simulink model "pd_path_sg"  (R2013b)
settings: Solver=ode45  StartTime=0.0  StopTime=10  RelTol=1e-3
undefined symbols (not defined in the file or in its folder): A, A2, B, C, D, EVAL, i, output_samp_bcoef, PCIN, reg_pk_lim, reg_plim, reg_scale, reg_sr_lim, reg_staclr, reg_txgain, THIS_DATE, W, X, Z
undefined symbols (not defined in the file): lut_address, lut_address_s5, reg_dltap
libraries: xbsIndex_r4 x3819, lut_ram_vhdl x32
(part 13 of 31)

== system pd_path_sg/A_lut_store/one_lut1/interp_a0 ==
  b0 : Inport
  b1 : Inport  Port=2
  delta : Inport  Port=3
  Convert : xbsIndex_r4/Convert  gui_display_data_type=Fixed-point  arith_type="Signed  (2's comp)"  n_bits=30  bin_pt=0  float_type=Single  exp_bits=8  fraction_bits=24  quantization=Truncate  overflow=Wrap  en=off  latency=0  pipeline=off  dbl_ovrd=off  block_type=convert
  Convert1 : xbsIndex_r4/Convert  gui_display_data_type=Fixed-point  arith_type="Signed  (2's comp)"  n_bits=48  bin_pt=0  float_type=Single  exp_bits=8  fraction_bits=24  quantization=Truncate  overflow=Wrap  en=off  latency=0  pipeline=off  dbl_ovrd=off  block_type=convert
  Convert2 : xbsIndex_r4/Convert  gui_display_data_type=Fixed-point  arith_type="Signed  (2's comp)"  n_bits=18  bin_pt=0  float_type=Single  exp_bits=8  fraction_bits=24  quantization=Truncate  overflow=Wrap  en=off  latency=0  pipeline=off  dbl_ovrd=off  block_type=convert
  Convert3 : xbsIndex_r4/Convert  gui_display_data_type=Fixed-point  arith_type="Signed  (2's comp)"  n_bits=27  bin_pt=0  float_type=Single  exp_bits=8  fraction_bits=24  quantization=Truncate  overflow=Wrap  en=off  latency=0  pipeline=off  dbl_ovrd=off  block_type=convert
  Convert4 : xbsIndex_r4/Convert  gui_display_data_type=Fixed-point  arith_type="Signed  (2's comp)"  n_bits=30  bin_pt=0  float_type=Single  exp_bits=8  fraction_bits=24  quantization=Truncate  overflow=Wrap  en=off  latency=0  pipeline=off  dbl_ovrd=off  block_type=convert
  Convert5 : xbsIndex_r4/Convert  gui_display_data_type=Fixed-point  arith_type="Signed  (2's comp)"  n_bits=18  bin_pt=0  float_type=Single  exp_bits=8  fraction_bits=24  quantization=Truncate  overflow=Wrap  en=off  latency=0  pipeline=off  dbl_ovrd=off  block_type=convert
  Convert6 : xbsIndex_r4/Convert  gui_display_data_type=Fixed-point  arith_type="Signed  (2's comp)"  n_bits=48  bin_pt=0  float_type=Single  exp_bits=8  fraction_bits=24  quantization=Truncate  overflow=Wrap  en=off  latency=0  pipeline=off  dbl_ovrd=off  block_type=convert
  Convert7 : xbsIndex_r4/Convert  gui_display_data_type=Fixed-point  arith_type="Signed  (2's comp)"  n_bits=27  bin_pt=0  float_type=Single  exp_bits=8  fraction_bits=24  quantization=Truncate  overflow=Wrap  en=off  latency=0  pipeline=off  dbl_ovrd=off  block_type=convert
  Convert8 : xbsIndex_r4/Convert  gui_display_data_type=Fixed-point  arith_type="Signed  (2's comp)"  n_bits=22  bin_pt=0  float_type=Single  exp_bits=8  fraction_bits=24  quantization=Truncate  overflow=Wrap  en=off  latency=0  pipeline=off  dbl_ovrd=off  block_type=convert
  Convert9 : xbsIndex_r4/Convert  gui_display_data_type=Fixed-point  arith_type="Signed  (2's comp)"  n_bits=22  bin_pt=0  float_type=Single  exp_bits=8  fraction_bits=24  quantization=Truncate  overflow=Wrap  en=off  latency=0  pipeline=off  dbl_ovrd=off  block_type=convert
  "DSP48E2 " : xbsIndex_r4/DSP48E2   use_a=Direct from A Port  use_b=Direct from B Port  addsub_mode=ONE48  xl_useadderonly=off  xl_dynamicmult=off  preaddinsel=A  amultsel=AD  bmultsel=B  enable_d=on  reset_preg=off  auto_reset_pr=RESET  pattern_from_creg=1  pattern='000000000000'  mask_from_creg=1  pattern_mask='000000000000'  rnd='000000000000'  widexor=off  xormode=1  use_op=on  use_creg=on  rst_all=off  en_all=off  use_pcin=off  use_carrycascin=off  use_multsignin=off  use_carryout=off  use_patterndetect=off  use_patternbdetect=off  use_overflow=off  use_underflow=off  use_acout=off  use_bcout=off  use_pcout=off  use_multsignout=off  use_carrycascout=off  pipeline_a=1  pipeline_b=2  pipeline_acout=1  pipeline_bcout=1  pipeline_c=on  pipeline_p=on  pipeline_mult=on  pipeline_opmode=on  pipeline_alumode=on  pipeline_carryin=on  pipeline_carryinsel=on  dreg=on  adreg=on  register_inmode=off  rst_a=off  rst_b=off  rst_c=off  rst_mult=off  rst_p=off  rst_carry_in=off  rst_alumode=off  rst_ctrl=off  reset_port_d=off  reset_port_inmode=off  en_a1=off  en_a2=off  en_b1=off  en_b2=off  en_c=off  en_mult=off  en_p=off  en_carry_in=off  en_alumode=off  en_multcarryin=off  en_ctrl=off  enable_port_regd=off  enable_port_regad=off  enable_port_reginmode=off  alumode_inverted=off  alumode_inverted_value='0000'  is_carryin_inverted=off  inmode_inverted=off  inmode_inverted_value='00000'  opmode_inverted=off  opmode_inverted_value='000000000'  is_rstallcarryin_inverted=off  is_rstalumode_inverted=off  is_rsta_inverted=off  is_rstb_inverted=off  is_rstc_inverted=off  is_rstd_inverted=off  is_rstctrl_inverted=off  is_rstinmode_inverted=off  is_rstm_inverted=off  is_rstp_inverted=off  use_synth_model=off  is_clk_inverted=false  block_type=dsp48e2
  DSP48E2 1 : xbsIndex_r4/DSP48E2   use_a=Direct from A Port  use_b=Direct from B Port  addsub_mode=ONE48  xl_useadderonly=off  xl_dynamicmult=off  preaddinsel=A  amultsel=AD  bmultsel=B  enable_d=on  reset_preg=off  auto_reset_pr=RESET  pattern_from_creg=1  pattern='000000000000'  mask_from_creg=1  pattern_mask='000000000000'  rnd='000000000000'  widexor=off  xormode=1  use_op=on  use_creg=on  rst_all=off  en_all=off  use_pcin=off  use_carrycascin=off  use_multsignin=off  use_carryout=off  use_patterndetect=off  use_patternbdetect=off  use_overflow=off  use_underflow=off  use_acout=off  use_bcout=off  use_pcout=off  use_multsignout=off  use_carrycascout=off  pipeline_a=1  pipeline_b=2  pipeline_acout=1  pipeline_bcout=1  pipeline_c=on  pipeline_p=on  pipeline_mult=on  pipeline_opmode=on  pipeline_alumode=on  pipeline_carryin=on  pipeline_carryinsel=on  dreg=on  adreg=on  register_inmode=off  rst_a=off  rst_b=off  rst_c=off  rst_mult=off  rst_p=off  rst_carry_in=off  rst_alumode=off  rst_ctrl=off  reset_port_d=off  reset_port_inmode=off  en_a1=off  en_a2=off  en_b1=off  en_b2=off  en_c=off  en_mult=off  en_p=off  en_carry_in=off  en_alumode=off  en_multcarryin=off  en_ctrl=off  enable_port_regd=off  enable_port_regad=off  enable_port_reginmode=off  alumode_inverted=off  alumode_inverted_value='0000'  is_carryin_inverted=off  inmode_inverted=off  inmode_inverted_value='00000'  opmode_inverted=off  opmode_inverted_value='000000000'  is_rstallcarryin_inverted=off  is_rstalumode_inverted=off  is_rsta_inverted=off  is_rstb_inverted=off  is_rstc_inverted=off  is_rstd_inverted=off  is_rstctrl_inverted=off  is_rstinmode_inverted=off  is_rstm_inverted=off  is_rstp_inverted=off  use_synth_model=off  is_clk_inverted=false  block_type=dsp48e2
  Delay : xbsIndex_r4/Delay  rst=off  infoeditControl=Selection of Reset will increase slice count due to use of real FFs and instead of SRLs  en=off  latency=2  reg_retiming=off  dbl_ovrd=off  block_type=delay
      settings: infoedit=Hardware notes: A delay line is a chain, each link of which is an SRL16 or SRL32 followed by a flip-flop.
  Delay1 : xbsIndex_r4/Delay  rst=off  infoeditControl=Selection of Reset will increase slice count due to use of real FFs and instead of SRLs  en=off  latency=2  reg_retiming=off  dbl_ovrd=off  block_type=delay
      settings: infoedit=Hardware notes: A delay line is a chain, each link of which is an SRL16 or SRL32 followed by a flip-flop.
  Delay2 : xbsIndex_r4/Delay  rst=off  infoeditControl=Selection of Reset will increase slice count due to use of real FFs and instead of SRLs  en=off  latency=1  reg_retiming=off  dbl_ovrd=off  block_type=delay
      settings: infoedit=Hardware notes: A delay line is a chain, each link of which is an SRL16 or SRL32 followed by a flip-flop.
  Delay3 : xbsIndex_r4/Delay  rst=off  infoeditControl=Selection of Reset will increase slice count due to use of real FFs and instead of SRLs  en=off  latency=1  reg_retiming=off  dbl_ovrd=off  block_type=delay
      settings: infoedit=Hardware notes: A delay line is a chain, each link of which is an SRL16 or SRL32 followed by a flip-flop.
  Demux : Demux  Outputs=2
  Demux1 : Demux  Outputs=2
  Mux : Mux  Inputs=2
  Opmode : xbsIndex_r4/Opmode  device=DSP48E2  equ=P=C+(A*B)  operation=C + A*B  inmode_0_3=D-A2  inmode_1_3=(D-A)*B  preaddinsel=A  amultsel=AD  bmultsel=B  inmode_0=A2  inmode_4=B2  logicinstr=X XOR Z  z_mux=PCIN>>17  xy_mux=P  w_mux=P  carry=CIN  dbl_ovrd=off  operand=+  x_mux=P  block_type=opmode
  Opmode1 : xbsIndex_r4/Opmode  device=DSP48E2  equ=P=C+(A*B)  operation=C + A*B  inmode_0_3=D-A2  inmode_1_3=(D-A)*B  preaddinsel=A  amultsel=AD  bmultsel=B  inmode_0=A2  inmode_4=B2  logicinstr=X XOR Z  z_mux=PCIN>>17  xy_mux=P  w_mux=P  carry=CIN  dbl_ovrd=off  operand=+  x_mux=P  block_type=opmode
  Reinterpret{,1..7} (8 alike) : xbsIndex_r4/Reinterpret  force_arith_type=on  arith_type="Signed  (2's comp)"  force_bin_pt=on  bin_pt=0  block_type=reinterpret
  Shift : xbsIndex_r4/Shift  shift_dir=Left  shift_bits=6  en=off  latency=0  precision=Full  arith_type="Signed  (2's comp)"  n_bits=16  bin_pt=14  quantization=Truncate  overflow=Wrap  dbl_ovrd=off  block_type=shift
  Shift1 : xbsIndex_r4/Shift  shift_dir=Left  shift_bits=6  en=off  latency=0  precision=Full  arith_type="Signed  (2's comp)"  n_bits=16  bin_pt=14  quantization=Truncate  overflow=Wrap  dbl_ovrd=off  block_type=shift
  q : Outport
  wires:
  Shift1/1 -> DSP48E2 1/3
  Shift/1 -> "DSP48E2 "/3
  Delay/1 -> Reinterpret1/1
  Delay1/1 -> Reinterpret6/1
  Mux/1 -> q/1
  "DSP48E2 "/1 -> Convert8/1
  Opmode1/1 -> "DSP48E2 "/5
  Convert7/1 -> "DSP48E2 "/4
  Reinterpret7/1 -> Convert7/1
  Convert6/1 -> Shift/1
  Reinterpret6/1 -> Convert6/1
  Convert5/1 -> "DSP48E2 "/2
  Reinterpret5/1 -> Convert5/1
  Convert4/1 -> "DSP48E2 "/1
  Reinterpret4/1 -> Convert4/1
  delta/1 -> Reinterpret2/1, Reinterpret5/1
  b1/1 -> Demux1/1
  b0/1 -> Demux/1
  Convert9/1 -> Delay3/1
  Reinterpret3/1 -> Convert3/1
  Convert3/1 -> DSP48E2 1/4
  Reinterpret2/1 -> Convert2/1
  Convert2/1 -> DSP48E2 1/2
  Reinterpret1/1 -> Convert1/1
  Convert1/1 -> Shift1/1
  Convert/1 -> DSP48E2 1/1
  Reinterpret/1 -> Convert/1
  Opmode/1 -> DSP48E2 1/5
  DSP48E2 1/1 -> Convert9/1
  Delay2/1 -> Mux/1  "I"
  Convert8/1 -> Delay2/1
  Delay3/1 -> Mux/2  "Q"
  Demux/1 -> Delay1/1, Reinterpret4/1
  Demux/2 -> Reinterpret/1, Delay/1
  Demux1/1 -> Reinterpret7/1
  Demux1/2 -> Reinterpret3/1

== system pd_path_sg/A_lut_store/one_lut1/interp_a1 ==
  b0 : Inport
  b1 : Inport  Port=2
  delta : Inport  Port=3
  Convert : xbsIndex_r4/Convert  gui_display_data_type=Fixed-point  arith_type="Signed  (2's comp)"  n_bits=30  bin_pt=0  float_type=Single  exp_bits=8  fraction_bits=24  quantization=Truncate  overflow=Wrap  en=off  latency=0  pipeline=off  dbl_ovrd=off  block_type=convert
  Convert1 : xbsIndex_r4/Convert  gui_display_data_type=Fixed-point  arith_type="Signed  (2's comp)"  n_bits=48  bin_pt=0  float_type=Single  exp_bits=8  fraction_bits=24  quantization=Truncate  overflow=Wrap  en=off  latency=0  pipeline=off  dbl_ovrd=off  block_type=convert
  Convert2 : xbsIndex_r4/Convert  gui_display_data_type=Fixed-point  arith_type="Signed  (2's comp)"  n_bits=18  bin_pt=0  float_type=Single  exp_bits=8  fraction_bits=24  quantization=Truncate  overflow=Wrap  en=off  latency=0  pipeline=off  dbl_ovrd=off  block_type=convert
  Convert3 : xbsIndex_r4/Convert  gui_display_data_type=Fixed-point  arith_type="Signed  (2's comp)"  n_bits=27  bin_pt=0  float_type=Single  exp_bits=8  fraction_bits=24  quantization=Truncate  overflow=Wrap  en=off  latency=0  pipeline=off  dbl_ovrd=off  block_type=convert
  Convert4 : xbsIndex_r4/Convert  gui_display_data_type=Fixed-point  arith_type="Signed  (2's comp)"  n_bits=30  bin_pt=0  float_type=Single  exp_bits=8  fraction_bits=24  quantization=Truncate  overflow=Wrap  en=off  latency=0  pipeline=off  dbl_ovrd=off  block_type=convert
  Convert5 : xbsIndex_r4/Convert  gui_display_data_type=Fixed-point  arith_type="Signed  (2's comp)"  n_bits=18  bin_pt=0  float_type=Single  exp_bits=8  fraction_bits=24  quantization=Truncate  overflow=Wrap  en=off  latency=0  pipeline=off  dbl_ovrd=off  block_type=convert
  Convert6 : xbsIndex_r4/Convert  gui_display_data_type=Fixed-point  arith_type="Signed  (2's comp)"  n_bits=48  bin_pt=0  float_type=Single  exp_bits=8  fraction_bits=24  quantization=Truncate  overflow=Wrap  en=off  latency=0  pipeline=off  dbl_ovrd=off  block_type=convert
  Convert7 : xbsIndex_r4/Convert  gui_display_data_type=Fixed-point  arith_type="Signed  (2's comp)"  n_bits=27  bin_pt=0  float_type=Single  exp_bits=8  fraction_bits=24  quantization=Truncate  overflow=Wrap  en=off  latency=0  pipeline=off  dbl_ovrd=off  block_type=convert
  Convert8 : xbsIndex_r4/Convert  gui_display_data_type=Fixed-point  arith_type="Signed  (2's comp)"  n_bits=22  bin_pt=0  float_type=Single  exp_bits=8  fraction_bits=24  quantization=Truncate  overflow=Wrap  en=off  latency=0  pipeline=off  dbl_ovrd=off  block_type=convert
  Convert9 : xbsIndex_r4/Convert  gui_display_data_type=Fixed-point  arith_type="Signed  (2's comp)"  n_bits=22  bin_pt=0  float_type=Single  exp_bits=8  fraction_bits=24  quantization=Truncate  overflow=Wrap  en=off  latency=0  pipeline=off  dbl_ovrd=off  block_type=convert
  "DSP48E2 " : xbsIndex_r4/DSP48E2   use_a=Direct from A Port  use_b=Direct from B Port  addsub_mode=ONE48  xl_useadderonly=off  xl_dynamicmult=off  preaddinsel=A  amultsel=AD  bmultsel=B  enable_d=on  reset_preg=off  auto_reset_pr=RESET  pattern_from_creg=1  pattern='000000000000'  mask_from_creg=1  pattern_mask='000000000000'  rnd='000000000000'  widexor=off  xormode=1  use_op=on  use_creg=on  rst_all=off  en_all=off  use_pcin=off  use_carrycascin=off  use_multsignin=off  use_carryout=off  use_patterndetect=off  use_patternbdetect=off  use_overflow=off  use_underflow=off  use_acout=off  use_bcout=off  use_pcout=off  use_multsignout=off  use_carrycascout=off  pipeline_a=1  pipeline_b=2  pipeline_acout=1  pipeline_bcout=1  pipeline_c=on  pipeline_p=on  pipeline_mult=on  pipeline_opmode=on  pipeline_alumode=on  pipeline_carryin=on  pipeline_carryinsel=on  dreg=on  adreg=on  register_inmode=off  rst_a=off  rst_b=off  rst_c=off  rst_mult=off  rst_p=off  rst_carry_in=off  rst_alumode=off  rst_ctrl=off  reset_port_d=off  reset_port_inmode=off  en_a1=off  en_a2=off  en_b1=off  en_b2=off  en_c=off  en_mult=off  en_p=off  en_carry_in=off  en_alumode=off  en_multcarryin=off  en_ctrl=off  enable_port_regd=off  enable_port_regad=off  enable_port_reginmode=off  alumode_inverted=off  alumode_inverted_value='0000'  is_carryin_inverted=off  inmode_inverted=off  inmode_inverted_value='00000'  opmode_inverted=off  opmode_inverted_value='000000000'  is_rstallcarryin_inverted=off  is_rstalumode_inverted=off  is_rsta_inverted=off  is_rstb_inverted=off  is_rstc_inverted=off  is_rstd_inverted=off  is_rstctrl_inverted=off  is_rstinmode_inverted=off  is_rstm_inverted=off  is_rstp_inverted=off  use_synth_model=off  is_clk_inverted=false  block_type=dsp48e2
  DSP48E2 1 : xbsIndex_r4/DSP48E2   use_a=Direct from A Port  use_b=Direct from B Port  addsub_mode=ONE48  xl_useadderonly=off  xl_dynamicmult=off  preaddinsel=A  amultsel=AD  bmultsel=B  enable_d=on  reset_preg=off  auto_reset_pr=RESET  pattern_from_creg=1  pattern='000000000000'  mask_from_creg=1  pattern_mask='000000000000'  rnd='000000000000'  widexor=off  xormode=1  use_op=on  use_creg=on  rst_all=off  en_all=off  use_pcin=off  use_carrycascin=off  use_multsignin=off  use_carryout=off  use_patterndetect=off  use_patternbdetect=off  use_overflow=off  use_underflow=off  use_acout=off  use_bcout=off  use_pcout=off  use_multsignout=off  use_carrycascout=off  pipeline_a=1  pipeline_b=2  pipeline_acout=1  pipeline_bcout=1  pipeline_c=on  pipeline_p=on  pipeline_mult=on  pipeline_opmode=on  pipeline_alumode=on  pipeline_carryin=on  pipeline_carryinsel=on  dreg=on  adreg=on  register_inmode=off  rst_a=off  rst_b=off  rst_c=off  rst_mult=off  rst_p=off  rst_carry_in=off  rst_alumode=off  rst_ctrl=off  reset_port_d=off  reset_port_inmode=off  en_a1=off  en_a2=off  en_b1=off  en_b2=off  en_c=off  en_mult=off  en_p=off  en_carry_in=off  en_alumode=off  en_multcarryin=off  en_ctrl=off  enable_port_regd=off  enable_port_regad=off  enable_port_reginmode=off  alumode_inverted=off  alumode_inverted_value='0000'  is_carryin_inverted=off  inmode_inverted=off  inmode_inverted_value='00000'  opmode_inverted=off  opmode_inverted_value='000000000'  is_rstallcarryin_inverted=off  is_rstalumode_inverted=off  is_rsta_inverted=off  is_rstb_inverted=off  is_rstc_inverted=off  is_rstd_inverted=off  is_rstctrl_inverted=off  is_rstinmode_inverted=off  is_rstm_inverted=off  is_rstp_inverted=off  use_synth_model=off  is_clk_inverted=false  block_type=dsp48e2
  Delay : xbsIndex_r4/Delay  rst=off  infoeditControl=Selection of Reset will increase slice count due to use of real FFs and instead of SRLs  en=off  latency=2  reg_retiming=off  dbl_ovrd=off  block_type=delay
      settings: infoedit=Hardware notes: A delay line is a chain, each link of which is an SRL16 or SRL32 followed by a flip-flop.
  Delay1 : xbsIndex_r4/Delay  rst=off  infoeditControl=Selection of Reset will increase slice count due to use of real FFs and instead of SRLs  en=off  latency=2  reg_retiming=off  dbl_ovrd=off  block_type=delay
      settings: infoedit=Hardware notes: A delay line is a chain, each link of which is an SRL16 or SRL32 followed by a flip-flop.
  Delay2 : xbsIndex_r4/Delay  rst=off  infoeditControl=Selection of Reset will increase slice count due to use of real FFs and instead of SRLs  en=off  latency=1  reg_retiming=off  dbl_ovrd=off  block_type=delay
      settings: infoedit=Hardware notes: A delay line is a chain, each link of which is an SRL16 or SRL32 followed by a flip-flop.
  Delay3 : xbsIndex_r4/Delay  rst=off  infoeditControl=Selection of Reset will increase slice count due to use of real FFs and instead of SRLs  en=off  latency=1  reg_retiming=off  dbl_ovrd=off  block_type=delay
      settings: infoedit=Hardware notes: A delay line is a chain, each link of which is an SRL16 or SRL32 followed by a flip-flop.
  Demux : Demux  Outputs=2
  Demux1 : Demux  Outputs=2
  Mux : Mux  Inputs=2
  Opmode : xbsIndex_r4/Opmode  device=DSP48E2  equ=P=C+(A*B)  operation=C + A*B  inmode_0_3=D-A2  inmode_1_3=(D-A)*B  preaddinsel=A  amultsel=AD  bmultsel=B  inmode_0=A2  inmode_4=B2  logicinstr=X XOR Z  z_mux=PCIN>>17  xy_mux=P  w_mux=P  carry=CIN  dbl_ovrd=off  operand=+  x_mux=P  block_type=opmode
  Opmode1 : xbsIndex_r4/Opmode  device=DSP48E2  equ=P=C+(A*B)  operation=C + A*B  inmode_0_3=D-A2  inmode_1_3=(D-A)*B  preaddinsel=A  amultsel=AD  bmultsel=B  inmode_0=A2  inmode_4=B2  logicinstr=X XOR Z  z_mux=PCIN>>17  xy_mux=P  w_mux=P  carry=CIN  dbl_ovrd=off  operand=+  x_mux=P  block_type=opmode
  Reinterpret{,1..7} (8 alike) : xbsIndex_r4/Reinterpret  force_arith_type=on  arith_type="Signed  (2's comp)"  force_bin_pt=on  bin_pt=0  block_type=reinterpret
  Shift : xbsIndex_r4/Shift  shift_dir=Left  shift_bits=6  en=off  latency=0  precision=Full  arith_type="Signed  (2's comp)"  n_bits=16  bin_pt=14  quantization=Truncate  overflow=Wrap  dbl_ovrd=off  block_type=shift
  Shift1 : xbsIndex_r4/Shift  shift_dir=Left  shift_bits=6  en=off  latency=0  precision=Full  arith_type="Signed  (2's comp)"  n_bits=16  bin_pt=14  quantization=Truncate  overflow=Wrap  dbl_ovrd=off  block_type=shift
  q : Outport
  wires:
  Demux1/2 -> Reinterpret3/1
  Demux1/1 -> Reinterpret7/1
  Demux/2 -> Delay/1, Reinterpret/1
  Demux/1 -> Reinterpret4/1, Delay1/1
  Delay3/1 -> Mux/2  "Q"
  Convert8/1 -> Delay2/1
  Delay2/1 -> Mux/1  "I"
  DSP48E2 1/1 -> Convert9/1
  Opmode/1 -> DSP48E2 1/5
  Reinterpret/1 -> Convert/1
  Convert/1 -> DSP48E2 1/1
  Convert1/1 -> Shift1/1
  Reinterpret1/1 -> Convert1/1
  Convert2/1 -> DSP48E2 1/2
  Reinterpret2/1 -> Convert2/1
  Convert3/1 -> DSP48E2 1/4
  Reinterpret3/1 -> Convert3/1
  Convert9/1 -> Delay3/1
  b0/1 -> Demux/1
  b1/1 -> Demux1/1
  delta/1 -> Reinterpret5/1, Reinterpret2/1
  Reinterpret4/1 -> Convert4/1
  Convert4/1 -> "DSP48E2 "/1
  Reinterpret5/1 -> Convert5/1
  Convert5/1 -> "DSP48E2 "/2
  Reinterpret6/1 -> Convert6/1
  Convert6/1 -> Shift/1
  Reinterpret7/1 -> Convert7/1
  Convert7/1 -> "DSP48E2 "/4
  Opmode1/1 -> "DSP48E2 "/5
  "DSP48E2 "/1 -> Convert8/1
  Mux/1 -> q/1
  Delay1/1 -> Reinterpret6/1
  Delay/1 -> Reinterpret1/1
  Shift/1 -> "DSP48E2 "/3
  Shift1/1 -> DSP48E2 1/3

== system pd_path_sg/A_lut_store/one_lut1/interp_b ==
  b0 : Inport
  b1 : Inport  Port=2
  delta : Inport  Port=3
  Convert : xbsIndex_r4/Convert  gui_display_data_type=Fixed-point  arith_type="Signed  (2's comp)"  n_bits=30  bin_pt=0  float_type=Single  exp_bits=8  fraction_bits=24  quantization=Truncate  overflow=Wrap  en=off  latency=0  pipeline=off  dbl_ovrd=off  block_type=convert
  Convert1 : xbsIndex_r4/Convert  gui_display_data_type=Fixed-point  arith_type="Signed  (2's comp)"  n_bits=48  bin_pt=0  float_type=Single  exp_bits=8  fraction_bits=24  quantization=Truncate  overflow=Wrap  en=off  latency=0  pipeline=off  dbl_ovrd=off  block_type=convert
  Convert10 : xbsIndex_r4/Convert  gui_display_data_type=Fixed-point  arith_type="Signed  (2's comp)"  n_bits=16  bin_pt=0  float_type=Single  exp_bits=8  fraction_bits=24  quantization=Truncate  overflow=Wrap  en=off  latency=0  pipeline=off  dbl_ovrd=off  block_type=convert
  Convert2 : xbsIndex_r4/Convert  gui_display_data_type=Fixed-point  arith_type="Signed  (2's comp)"  n_bits=18  bin_pt=0  float_type=Single  exp_bits=8  fraction_bits=24  quantization=Truncate  overflow=Wrap  en=off  latency=0  pipeline=off  dbl_ovrd=off  block_type=convert
  Convert3 : xbsIndex_r4/Convert  gui_display_data_type=Fixed-point  arith_type="Signed  (2's comp)"  n_bits=27  bin_pt=0  float_type=Single  exp_bits=8  fraction_bits=24  quantization=Truncate  overflow=Wrap  en=off  latency=0  pipeline=off  dbl_ovrd=off  block_type=convert
  Convert4 : xbsIndex_r4/Convert  gui_display_data_type=Fixed-point  arith_type="Signed  (2's comp)"  n_bits=30  bin_pt=0  float_type=Single  exp_bits=8  fraction_bits=24  quantization=Truncate  overflow=Wrap  en=off  latency=0  pipeline=off  dbl_ovrd=off  block_type=convert
  Convert5 : xbsIndex_r4/Convert  gui_display_data_type=Fixed-point  arith_type="Signed  (2's comp)"  n_bits=18  bin_pt=0  float_type=Single  exp_bits=8  fraction_bits=24  quantization=Truncate  overflow=Wrap  en=off  latency=0  pipeline=off  dbl_ovrd=off  block_type=convert
  Convert6 : xbsIndex_r4/Convert  gui_display_data_type=Fixed-point  arith_type="Signed  (2's comp)"  n_bits=48  bin_pt=0  float_type=Single  exp_bits=8  fraction_bits=24  quantization=Truncate  overflow=Wrap  en=off  latency=0  pipeline=off  dbl_ovrd=off  block_type=convert
  Convert7 : xbsIndex_r4/Convert  gui_display_data_type=Fixed-point  arith_type="Signed  (2's comp)"  n_bits=27  bin_pt=0  float_type=Single  exp_bits=8  fraction_bits=24  quantization=Truncate  overflow=Wrap  en=off  latency=0  pipeline=off  dbl_ovrd=off  block_type=convert
  Convert8 : xbsIndex_r4/Convert  gui_display_data_type=Fixed-point  arith_type="Signed  (2's comp)"  n_bits=16  bin_pt=0  float_type=Single  exp_bits=8  fraction_bits=24  quantization=Truncate  overflow=Wrap  en=off  latency=0  pipeline=off  dbl_ovrd=off  block_type=convert
  "DSP48E2 " : xbsIndex_r4/DSP48E2   use_a=Direct from A Port  use_b=Direct from B Port  addsub_mode=ONE48  xl_useadderonly=off  xl_dynamicmult=off  preaddinsel=A  amultsel=AD  bmultsel=B  enable_d=on  reset_preg=off  auto_reset_pr=RESET  pattern_from_creg=1  pattern='000000000000'  mask_from_creg=1  pattern_mask='000000000000'  rnd='000000000800'  widexor=off  xormode=1  use_op=on  use_creg=on  rst_all=off  en_all=off  use_pcin=off  use_carrycascin=off  use_multsignin=off  use_carryout=off  use_patterndetect=off  use_patternbdetect=off  use_overflow=off  use_underflow=off  use_acout=off  use_bcout=off  use_pcout=off  use_multsignout=off  use_carrycascout=off  pipeline_a=1  pipeline_b=2  pipeline_acout=1  pipeline_bcout=1  pipeline_c=on  pipeline_p=on  pipeline_mult=on  pipeline_opmode=on  pipeline_alumode=on  pipeline_carryin=on  pipeline_carryinsel=on  dreg=on  adreg=on  register_inmode=off  rst_a=off  rst_b=off  rst_c=off  rst_mult=off  rst_p=off  rst_carry_in=off  rst_alumode=off  rst_ctrl=off  reset_port_d=off  reset_port_inmode=off  en_a1=off  en_a2=off  en_b1=off  en_b2=off  en_c=off  en_mult=off  en_p=off  en_carry_in=off  en_alumode=off  en_multcarryin=off  en_ctrl=off  enable_port_regd=off  enable_port_regad=off  enable_port_reginmode=off  alumode_inverted=off  alumode_inverted_value='0000'  is_carryin_inverted=off  inmode_inverted=off  inmode_inverted_value='00000'  opmode_inverted=off  opmode_inverted_value='000000000'  is_rstallcarryin_inverted=off  is_rstalumode_inverted=off  is_rsta_inverted=off  is_rstb_inverted=off  is_rstc_inverted=off  is_rstd_inverted=off  is_rstctrl_inverted=off  is_rstinmode_inverted=off  is_rstm_inverted=off  is_rstp_inverted=off  use_synth_model=off  is_clk_inverted=false  block_type=dsp48e2
  DSP48E2 1 : xbsIndex_r4/DSP48E2   use_a=Direct from A Port  use_b=Direct from B Port  addsub_mode=ONE48  xl_useadderonly=off  xl_dynamicmult=off  preaddinsel=A  amultsel=AD  bmultsel=B  enable_d=on  reset_preg=off  auto_reset_pr=RESET  pattern_from_creg=1  pattern='000000000000'  mask_from_creg=1  pattern_mask='000000000000'  rnd='000000000800'  widexor=off  xormode=1  use_op=on  use_creg=on  rst_all=off  en_all=off  use_pcin=off  use_carrycascin=off  use_multsignin=off  use_carryout=off  use_patterndetect=off  use_patternbdetect=off  use_overflow=off  use_underflow=off  use_acout=off  use_bcout=off  use_pcout=off  use_multsignout=off  use_carrycascout=off  pipeline_a=1  pipeline_b=2  pipeline_acout=1  pipeline_bcout=1  pipeline_c=on  pipeline_p=on  pipeline_mult=on  pipeline_opmode=on  pipeline_alumode=on  pipeline_carryin=on  pipeline_carryinsel=on  dreg=on  adreg=on  register_inmode=off  rst_a=off  rst_b=off  rst_c=off  rst_mult=off  rst_p=off  rst_carry_in=off  rst_alumode=off  rst_ctrl=off  reset_port_d=off  reset_port_inmode=off  en_a1=off  en_a2=off  en_b1=off  en_b2=off  en_c=off  en_mult=off  en_p=off  en_carry_in=off  en_alumode=off  en_multcarryin=off  en_ctrl=off  enable_port_regd=off  enable_port_regad=off  enable_port_reginmode=off  alumode_inverted=off  alumode_inverted_value='0000'  is_carryin_inverted=off  inmode_inverted=off  inmode_inverted_value='00000'  opmode_inverted=off  opmode_inverted_value='000000000'  is_rstallcarryin_inverted=off  is_rstalumode_inverted=off  is_rsta_inverted=off  is_rstb_inverted=off  is_rstc_inverted=off  is_rstd_inverted=off  is_rstctrl_inverted=off  is_rstinmode_inverted=off  is_rstm_inverted=off  is_rstp_inverted=off  use_synth_model=off  is_clk_inverted=false  block_type=dsp48e2
  Delay : xbsIndex_r4/Delay  rst=off  infoeditControl=Selection of Reset will increase slice count due to use of real FFs and instead of SRLs  en=off  latency=2  reg_retiming=off  dbl_ovrd=off  block_type=delay
      settings: infoedit=Hardware notes: A delay line is a chain, each link of which is an SRL16 or SRL32 followed by a flip-flop.
  Delay1 : xbsIndex_r4/Delay  rst=off  infoeditControl=Selection of Reset will increase slice count due to use of real FFs and instead of SRLs  en=off  latency=2  reg_retiming=off  dbl_ovrd=off  block_type=delay
      settings: infoedit=Hardware notes: A delay line is a chain, each link of which is an SRL16 or SRL32 followed by a flip-flop.
  Delay2 : xbsIndex_r4/Delay  rst=off  infoeditControl=Selection of Reset will increase slice count due to use of real FFs and instead of SRLs  en=off  latency=1  reg_retiming=off  dbl_ovrd=off  block_type=delay
  Delay3 : xbsIndex_r4/Delay  rst=off  infoeditControl=Selection of Reset will increase slice count due to use of real FFs and instead of SRLs  en=off  latency=1  reg_retiming=off  dbl_ovrd=off  block_type=delay
  Demux : Demux  Outputs=2
  Demux1 : Demux  Outputs=2
  Mux : Mux  Inputs=2
  Opmode1 : xbsIndex_r4/Opmode  device=DSP48E2  equ=P=C+(A*B)+RND  operation=Custom  inmode_0_3=D+A2  inmode_1_3=(D-A)*B  preaddinsel=A  amultsel=AD  bmultsel=B  inmode_0=A2  inmode_4=B2  logicinstr=X + W + Z  z_mux=C  xy_mux=A*B  w_mux=RND  carry=0  dbl_ovrd=off  operand=+  x_mux=P  block_type=opmode
  Opmode2 : xbsIndex_r4/Opmode  device=DSP48E2  equ=P=C+(A*B)+RND  operation=Custom  inmode_0_3=D+A2  inmode_1_3=(D-A)*B  preaddinsel=A  amultsel=AD  bmultsel=B  inmode_0=A2  inmode_4=B2  logicinstr=X + W + Z  z_mux=C  xy_mux=A*B  w_mux=RND  carry=0  dbl_ovrd=off  operand=+  x_mux=P  block_type=opmode
  Reinterpret{,1..7} (8 alike) : xbsIndex_r4/Reinterpret  force_arith_type=on  arith_type="Signed  (2's comp)"  force_bin_pt=on  bin_pt=0  block_type=reinterpret
  Shift : xbsIndex_r4/Shift  shift_dir=Left  shift_bits=6  en=off  latency=0  precision=Full  arith_type="Signed  (2's comp)"  n_bits=16  bin_pt=14  quantization=Truncate  overflow=Wrap  dbl_ovrd=off  block_type=shift
  Shift1 : xbsIndex_r4/Shift  shift_dir=Left  shift_bits=6  en=off  latency=0  precision=Full  arith_type="Signed  (2's comp)"  n_bits=16  bin_pt=14  quantization=Truncate  overflow=Wrap  dbl_ovrd=off  block_type=shift
  Slice1 : xbsIndex_r4/Slice  nbits=16  boolean_output=off  mode=Lower Bit Location + Width  bit1=0  base1=MSB of Input  bit0=12  base0=LSB of Input  dbl_ovrd=off  block_type=slice
  Slice2 : xbsIndex_r4/Slice  nbits=16  boolean_output=off  mode=Lower Bit Location + Width  bit1=0  base1=MSB of Input  bit0=12  base0=LSB of Input  dbl_ovrd=off  block_type=slice
  q : Outport
  wires:
  DSP48E2 1/1 -> Slice1/1
  Opmode1/1 -> DSP48E2 1/5
  Reinterpret/1 -> Convert/1
  Convert/1 -> DSP48E2 1/1
  Convert1/1 -> Shift1/1
  Reinterpret1/1 -> Convert1/1
  Convert2/1 -> DSP48E2 1/2
  Reinterpret2/1 -> Convert2/1
  Convert3/1 -> DSP48E2 1/4
  Reinterpret3/1 -> Convert3/1
  Delay3/1 -> Mux/2  "Q"
  b0/1 -> Demux/1
  b1/1 -> Demux1/1
  Demux/1 -> Reinterpret4/1, Delay1/1
  Demux1/1 -> Reinterpret7/1
  delta/1 -> Reinterpret5/1, Reinterpret2/1
  Demux1/2 -> Reinterpret3/1
  Demux/2 -> Delay/1, Reinterpret/1
  Reinterpret4/1 -> Convert4/1
  Convert4/1 -> "DSP48E2 "/1
  Reinterpret5/1 -> Convert5/1
  Convert5/1 -> "DSP48E2 "/2
  Reinterpret6/1 -> Convert6/1
  Convert6/1 -> Shift/1
  Reinterpret7/1 -> Convert7/1
  Convert7/1 -> "DSP48E2 "/4
  Opmode2/1 -> "DSP48E2 "/5
  Delay2/1 -> Mux/1  "I"
  Mux/1 -> q/1
  Delay1/1 -> Reinterpret6/1
  Delay/1 -> Reinterpret1/1
  Shift/1 -> "DSP48E2 "/3
  Shift1/1 -> DSP48E2 1/3
  Slice2/1 -> Convert10/1
  "DSP48E2 "/1 -> Slice2/1
  Convert10/1 -> Delay2/1
  Slice1/1 -> Convert8/1
  Convert8/1 -> Delay3/1

== system pd_path_sg/A_lut_store/one_lut1/iqslice ==
  d32 : Inport
  Convert1 : xbsIndex_r4/Convert  gui_display_data_type=Fixed-point  arith_type="Signed  (2's comp)"  n_bits=16  bin_pt=0  float_type=Single  exp_bits=8  fraction_bits=24  quantization=Truncate  overflow=Wrap  en=off  latency=0  pipeline=off  dbl_ovrd=off  block_type=convert
  Convert9 : xbsIndex_r4/Convert  gui_display_data_type=Fixed-point  arith_type="Signed  (2's comp)"  n_bits=16  bin_pt=0  float_type=Single  exp_bits=8  fraction_bits=24  quantization=Truncate  overflow=Wrap  en=off  latency=0  pipeline=off  dbl_ovrd=off  block_type=convert
  Delay1 : xbsIndex_r4/Delay  rst=off  infoeditControl=Selection of Reset will increase slice count due to use of real FFs and instead of SRLs  en=off  latency=1  reg_retiming=off  dbl_ovrd=off  block_type=delay
      settings: infoedit=Hardware notes: A delay line is a chain, each link of which is an SRL16 or SRL32 followed by a flip-flop.
  Mux1 : Mux  Inputs=2
  Slice : xbsIndex_r4/Slice  nbits=16  boolean_output=off  mode=Lower Bit Location + Width  bit1=0  base1=MSB of Input  bit0=0  base0=LSB of Input  dbl_ovrd=off  block_type=slice
  Slice1 : xbsIndex_r4/Slice  nbits=16  boolean_output=off  mode=Lower Bit Location + Width  bit1=0  base1=MSB of Input  bit0=16  base0=LSB of Input  dbl_ovrd=off  block_type=slice
  ciq : Outport
  wires:
  Delay1/1 -> Slice/1, Slice1/1
  Slice1/1 -> Convert1/1
  Slice/1 -> Convert9/1
  d32/1 -> Delay1/1
  Mux1/1 -> ciq/1
  Convert9/1 -> Mux1/1
  Convert1/1 -> Mux1/2

== system pd_path_sg/A_lut_store/one_lut1/iqslice1 ==
  d32 : Inport
  Convert1 : xbsIndex_r4/Convert  gui_display_data_type=Fixed-point  arith_type="Signed  (2's comp)"  n_bits=16  bin_pt=0  float_type=Single  exp_bits=8  fraction_bits=24  quantization=Truncate  overflow=Wrap  en=off  latency=0  pipeline=off  dbl_ovrd=off  block_type=convert
  Convert9 : xbsIndex_r4/Convert  gui_display_data_type=Fixed-point  arith_type="Signed  (2's comp)"  n_bits=16  bin_pt=0  float_type=Single  exp_bits=8  fraction_bits=24  quantization=Truncate  overflow=Wrap  en=off  latency=0  pipeline=off  dbl_ovrd=off  block_type=convert
  Delay1 : xbsIndex_r4/Delay  rst=off  infoeditControl=Selection of Reset will increase slice count due to use of real FFs and instead of SRLs  en=off  latency=1  reg_retiming=off  dbl_ovrd=off  block_type=delay
      settings: infoedit=Hardware notes: A delay line is a chain, each link of which is an SRL16 or SRL32 followed by a flip-flop.
  Mux1 : Mux  Inputs=2
  Slice : xbsIndex_r4/Slice  nbits=16  boolean_output=off  mode=Lower Bit Location + Width  bit1=0  base1=MSB of Input  bit0=0  base0=LSB of Input  dbl_ovrd=off  block_type=slice
  Slice1 : xbsIndex_r4/Slice  nbits=16  boolean_output=off  mode=Lower Bit Location + Width  bit1=0  base1=MSB of Input  bit0=16  base0=LSB of Input  dbl_ovrd=off  block_type=slice
  ciq : Outport
  wires:
  Convert1/1 -> Mux1/2
  Convert9/1 -> Mux1/1
  Mux1/1 -> ciq/1
  d32/1 -> Delay1/1
  Slice/1 -> Convert9/1
  Slice1/1 -> Convert1/1
  Delay1/1 -> Slice1/1, Slice/1

== system pd_path_sg/A_lut_store/one_lut1/iqslice2 ==
  d32 : Inport
  Convert1 : xbsIndex_r4/Convert  gui_display_data_type=Fixed-point  arith_type="Signed  (2's comp)"  n_bits=16  bin_pt=0  float_type=Single  exp_bits=8  fraction_bits=24  quantization=Truncate  overflow=Wrap  en=off  latency=0  pipeline=off  dbl_ovrd=off  block_type=convert
  Convert9 : xbsIndex_r4/Convert  gui_display_data_type=Fixed-point  arith_type="Signed  (2's comp)"  n_bits=16  bin_pt=0  float_type=Single  exp_bits=8  fraction_bits=24  quantization=Truncate  overflow=Wrap  en=off  latency=0  pipeline=off  dbl_ovrd=off  block_type=convert
  Delay1 : xbsIndex_r4/Delay  rst=off  infoeditControl=Selection of Reset will increase slice count due to use of real FFs and instead of SRLs  en=off  latency=1  reg_retiming=off  dbl_ovrd=off  block_type=delay
      settings: infoedit=Hardware notes: A delay line is a chain, each link of which is an SRL16 or SRL32 followed by a flip-flop.
  Mux1 : Mux  Inputs=2
  Slice : xbsIndex_r4/Slice  nbits=16  boolean_output=off  mode=Lower Bit Location + Width  bit1=0  base1=MSB of Input  bit0=0  base0=LSB of Input  dbl_ovrd=off  block_type=slice
  Slice1 : xbsIndex_r4/Slice  nbits=16  boolean_output=off  mode=Lower Bit Location + Width  bit1=0  base1=MSB of Input  bit0=16  base0=LSB of Input  dbl_ovrd=off  block_type=slice
  ciq : Outport
  wires:
  Delay1/1 -> Slice/1, Slice1/1
  Slice1/1 -> Convert1/1
  Slice/1 -> Convert9/1
  d32/1 -> Delay1/1
  Mux1/1 -> ciq/1
  Convert9/1 -> Mux1/1
  Convert1/1 -> Mux1/2

== system pd_path_sg/A_lut_store/one_lut1/iqslice3 ==
  d32 : Inport
  Convert1 : xbsIndex_r4/Convert  gui_display_data_type=Fixed-point  arith_type="Signed  (2's comp)"  n_bits=16  bin_pt=0  float_type=Single  exp_bits=8  fraction_bits=24  quantization=Truncate  overflow=Wrap  en=off  latency=0  pipeline=off  dbl_ovrd=off  block_type=convert
  Convert9 : xbsIndex_r4/Convert  gui_display_data_type=Fixed-point  arith_type="Signed  (2's comp)"  n_bits=16  bin_pt=0  float_type=Single  exp_bits=8  fraction_bits=24  quantization=Truncate  overflow=Wrap  en=off  latency=0  pipeline=off  dbl_ovrd=off  block_type=convert
  Delay1 : xbsIndex_r4/Delay  rst=off  infoeditControl=Selection of Reset will increase slice count due to use of real FFs and instead of SRLs  en=off  latency=1  reg_retiming=off  dbl_ovrd=off  block_type=delay
      settings: infoedit=Hardware notes: A delay line is a chain, each link of which is an SRL16 or SRL32 followed by a flip-flop.
  Mux1 : Mux  Inputs=2
  Slice : xbsIndex_r4/Slice  nbits=16  boolean_output=off  mode=Lower Bit Location + Width  bit1=0  base1=MSB of Input  bit0=0  base0=LSB of Input  dbl_ovrd=off  block_type=slice
  Slice1 : xbsIndex_r4/Slice  nbits=16  boolean_output=off  mode=Lower Bit Location + Width  bit1=0  base1=MSB of Input  bit0=16  base0=LSB of Input  dbl_ovrd=off  block_type=slice
  ciq : Outport
  wires:
  Convert1/1 -> Mux1/2
  Convert9/1 -> Mux1/1
  Mux1/1 -> ciq/1
  d32/1 -> Delay1/1
  Slice/1 -> Convert9/1
  Slice1/1 -> Convert1/1
  Delay1/1 -> Slice1/1, Slice/1

== system pd_path_sg/A_lut_store/one_lut1/split_if1 ==
  d : Inport
  frac : xbsIndex_r4/Slice  nbits=6  boolean_output=off  mode=Lower Bit Location + Width  bit1=0  base1=MSB of Input  bit0=0  base0=LSB of Input  dbl_ovrd=off  block_type=slice
  integer : xbsIndex_r4/Slice  nbits=4  boolean_output=off  mode=Lower Bit Location + Width  bit1=0  base1=MSB of Input  bit0=6  base0=LSB of Input  dbl_ovrd=off  block_type=slice
  iaddr : Outport
  faddr : Outport  Port=2
  wires:
  frac/1 -> faddr/1
  integer/1 -> iaddr/1
  d/1 -> frac/1, integer/1

== system pd_path_sg/A_lut_store/one_lut1/split_if2 ==
  d : Inport
  frac : xbsIndex_r4/Slice  nbits=6  boolean_output=off  mode=Lower Bit Location + Width  bit1=0  base1=MSB of Input  bit0=0  base0=LSB of Input  dbl_ovrd=off  block_type=slice
  integer : xbsIndex_r4/Slice  nbits=4  boolean_output=off  mode=Lower Bit Location + Width  bit1=0  base1=MSB of Input  bit0=6  base0=LSB of Input  dbl_ovrd=off  block_type=slice
  iaddr : Outport
  faddr : Outport  Port=2
  wires:
  d/1 -> integer/1, frac/1
  integer/1 -> iaddr/1
  frac/1 -> faddr/1

== system pd_path_sg/A_lut_store/one_lut2/B ==
  d : Inport
  Delay : xbsIndex_r4/Delay  rst=off  infoeditControl=Selection of Reset will increase slice count due to use of real FFs and instead of SRLs  en=off  latency=1  reg_retiming=off  dbl_ovrd=off  block_type=delay
      settings: infoedit=Hardware notes: A delay line is a chain, each link of which is an SRL16 or SRL32 followed by a flip-flop.
  Slice : xbsIndex_r4/Slice  nbits=3  boolean_output=off  mode=Lower Bit Location + Width  bit1=0  base1=MSB of Input  bit0=1  base0=LSB of Input  dbl_ovrd=off  block_type=slice
  q : Outport
  wires:
  d/1 -> Delay/1
  Slice/1 -> q/1
  Delay/1 -> Slice/1

== system pd_path_sg/A_lut_store/one_lut2/Bf ==
  iaddr : Inport
  delta : Inport  Port=2
  AddSub : xbsIndex_r4/AddSub  mode=Subtraction  use_carryin=off  use_carryout=off  en=off  latency=0  precision=Full  arith_type=Unsigned  n_bits=16  bin_pt=14  quantization=Truncate  overflow=Wrap  use_behavioral_HDL=off  hw_selection=Fabric  pipelined=off  dbl_ovrd=off  block_type=addsub
  Constant : xbsIndex_r4/Constant  const=1.0  gui_display_data_type=Fixed-point  arith_type=Unsigned  n_bits=6  bin_pt=5  preci_type=Single  exp_width=8  frac_width=24  explicit_period=off  period=1  equ=P=C  opselect=C  inp2=PCIN>>17  opr=+  inp1=P  carry=CIN  dbl_ovrd=off  block_type=constant
  Convert : xbsIndex_r4/Convert  gui_display_data_type=Fixed-point  arith_type=Unsigned  n_bits=6  bin_pt=6  float_type=Single  exp_bits=8  fraction_bits=24  quantization=Truncate  overflow=Wrap  en=off  latency=0  pipeline=off  dbl_ovrd=off  block_type=convert
  Mux : xbsIndex_r4/Mux  inputs=2  en=off  latency=1  precision=Full  arith_type=Unsigned  n_bits=16  bin_pt=14  quantization=Truncate  overflow=Wrap  dbl_ovrd=off  block_type=mux
  Reinterpret : xbsIndex_r4/Reinterpret  force_arith_type=on  arith_type=Unsigned  force_bin_pt=on  bin_pt=6  block_type=reinterpret
  Slice : xbsIndex_r4/Slice  nbits=1  boolean_output=off  mode=Lower Bit Location + Width  bit1=0  base1=MSB of Input  bit0=0  base0=LSB of Input  dbl_ovrd=off  block_type=slice
  q : Outport
  wires:
  iaddr/1 -> Slice/1
  AddSub/1 -> Mux/3
  Mux/1 -> q/1
  Constant/1 -> AddSub/1
  delta/1 -> Reinterpret/1
  Slice/1 -> Mux/1
  Reinterpret/1 -> Convert/1
  Convert/1 -> AddSub/2, Mux/2

== system pd_path_sg/A_lut_store/one_lut2/Bp1 ==
  d : Inport
  AddSub : xbsIndex_r4/AddSub  mode=Addition  use_carryin=off  use_carryout=off  en=off  latency=1  precision=Full  arith_type=Unsigned  n_bits=16  bin_pt=14  quantization=Truncate  overflow=Wrap  use_behavioral_HDL=off  hw_selection=Fabric  pipelined=off  dbl_ovrd=off  block_type=addsub
  Constant : xbsIndex_r4/Constant  const=1.0  gui_display_data_type=Fixed-point  arith_type=Unsigned  n_bits=4  bin_pt=0  preci_type=Single  exp_width=8  frac_width=24  explicit_period=off  period=1  equ=P=C  opselect=C  inp2=PCIN>>17  opr=+  inp1=P  carry=CIN  dbl_ovrd=off  block_type=constant
  Slice : xbsIndex_r4/Slice  nbits=3  boolean_output=off  mode=Lower Bit Location + Width  bit1=0  base1=MSB of Input  bit0=1  base0=LSB of Input  dbl_ovrd=off  block_type=slice
  q : Outport
  wires:
  d/1 -> AddSub/1
  Constant/1 -> AddSub/2
  AddSub/1 -> Slice/1
  Slice/1 -> q/1

== system pd_path_sg/A_lut_store/one_lut2/addr_gen ==
  chn : Inport
  active0 : Inport  Port=2
  active1 : Inport  Port=3
  addr0 : Inport  Port=4
  addr1 : Inport  Port=5
  Concat : xbsIndex_r4/Concat  num_inputs=3  dbl_ovrd=off  block_type=concat
  Concat1 : xbsIndex_r4/Concat  num_inputs=3  dbl_ovrd=off  block_type=concat
  Delay : xbsIndex_r4/Delay  rst=off  infoeditControl=Selection of Reset will increase slice count due to use of real FFs and instead of SRLs  en=off  latency=1  reg_retiming=off  dbl_ovrd=off  block_type=delay
      settings: infoedit=Hardware notes: A delay line is a chain, each link of which is an SRL16 or SRL32 followed by a flip-flop.
  Delay1 : xbsIndex_r4/Delay  rst=off  infoeditControl=Selection of Reset will increase slice count due to use of real FFs and instead of SRLs  en=off  latency=1  reg_retiming=off  dbl_ovrd=off  block_type=delay
      settings: infoedit=Hardware notes: A delay line is a chain, each link of which is an SRL16 or SRL32 followed by a flip-flop.
  Mux : xbsIndex_r4/Mux  inputs=2  en=off  latency=1  precision=Full  arith_type=Unsigned  n_bits=16  bin_pt=14  quantization=Truncate  overflow=Wrap  dbl_ovrd=off  block_type=mux
  Mux1 : xbsIndex_r4/Mux  inputs=2  en=off  latency=1  precision=Full  arith_type=Unsigned  n_bits=16  bin_pt=14  quantization=Truncate  overflow=Wrap  dbl_ovrd=off  block_type=mux
  rd_addr0 : Outport
  rd_addr1 : Outport  Port=2
  wires:
  addr1/1 -> Concat1/3
  Concat1/1 -> rd_addr1/1
  Concat/1 -> rd_addr0/1  "rd_addr"
  addr0/1 -> Concat/3
  Delay/1 -> Concat/1
  Mux/1 -> Concat/2
  chn/1 -> Mux1/1, Delay1/1, Mux/1, Delay/1
  active0/1 -> Mux1/2, Mux/2
  active1/1 -> Mux1/3, Mux/3
  Mux1/1 -> Concat1/2
  Delay1/1 -> Concat1/1
